simulink model "project4_week2"  (R2020b)
settings: Solver=VariableStepAuto  StartTime=0.0  StopTime=10.0  RelTol=1e-3
undefined symbols (not defined in the file): b, J, K, kd, ki, kp, L, n, R
settings Model: Creator=RASIKA MALGI  LastModifiedBy=RASIKA MALGI

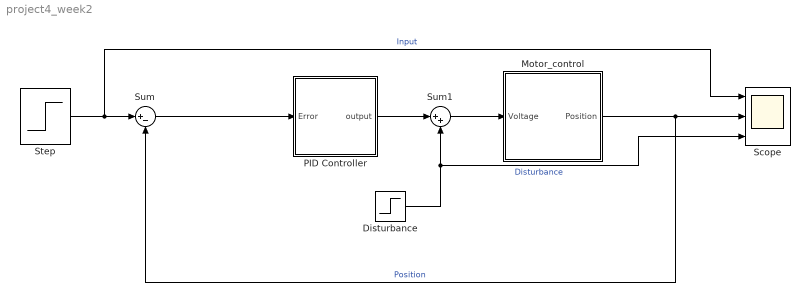
== system project4_week2 ==
  Disturbance : Step  Time=0.06  SampleTime=0
  Motor_control : Subsystem
  PID Controller : Subsystem  TreatAsAtomicUnit=on
  Scope : Scope  NumInputPorts=3
  Step : Step  Time=0  SampleTime=0
  Sum : Sum  Inputs=|+-
  Sum1 : Sum  Inputs=|++
  wires:
  PID Controller/1(output) -> Sum1/1
  Motor_control/1(Position) -> Sum/2, Scope/2  "Position"
  Step/1 -> Scope/1, Sum/1  "Input"
  Disturbance/1 -> Scope/3, Sum1/2  "Disturbance"
  Sum/1 -> PID Controller/1(Error)
  Sum1/1 -> Motor_control/1(Voltage)

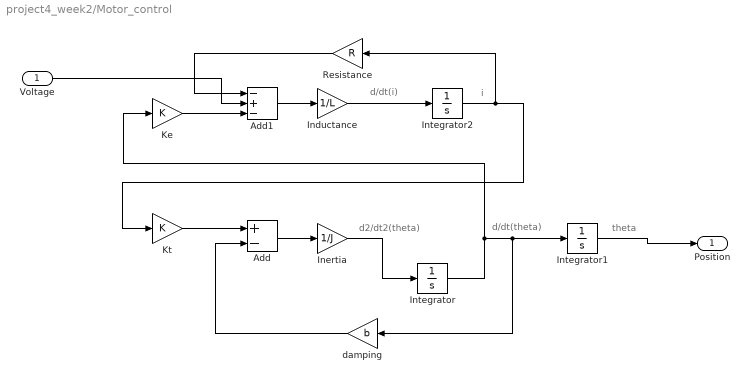
== system project4_week2/Motor_control ==
  note: i
  note: d/dt(i)
  note: theta
  note: d/dt(theta)
  note: d2/dt2(theta)
  Voltage : Inport
  Add : Sum  Inputs=+-
  Add1 : Sum  Inputs=-+-
  Inductance : Gain  Gain=1/L
  Inertia : Gain  Gain=1/J
  Integrator : Integrator
  Integrator1 : Integrator
  Integrator2 : Integrator
  Ke : Gain  Gain=K
  Kt : Gain  Gain=K
  Resistance : Gain  Gain=R
  damping : Gain  Gain=b
  Position : Outport
  wires:
  Add/1 -> Inertia/1
  Inductance/1 -> Integrator2/1
  Add1/1 -> Inductance/1
  Ke/1 -> Add1/3
  Integrator/1 -> Ke/1, damping/1, Integrator1/1
  damping/1 -> Add/2
  Inertia/1 -> Integrator/1
  Kt/1 -> Add/1
  Integrator2/1 -> Resistance/1, Kt/1
  Resistance/1 -> Add1/1
  Voltage/1 -> Add1/2
  Integrator1/1 -> Position/1

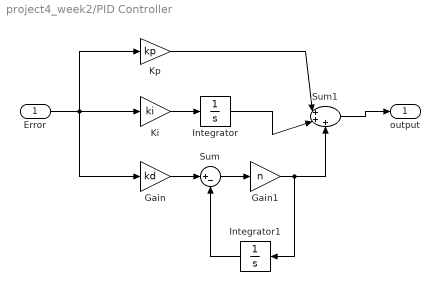
== system project4_week2/PID Controller ==
  Error : Inport
  Gain : Gain  Gain=kd
  Gain1 : Gain  Gain=n
  Integrator : Integrator
  Integrator1 : Integrator
  Ki : Gain  Gain=ki
  Kp : Gain  Gain=kp
  Sum : Sum  Inputs=|+-
  Sum1 : Sum  Inputs=|+++
  output : Outport
  wires:
  Error/1 -> Gain/1, Ki/1, Kp/1
  Sum1/1 -> output/1
  Kp/1 -> Sum1/1
  Ki/1 -> Integrator/1
  Integrator/1 -> Sum1/2
  Gain/1 -> Sum/1
  Sum/1 -> Gain1/1
  Gain1/1 -> Integrator1/1, Sum1/3
  Integrator1/1 -> Sum/2
